simulink model "FOC_Compatible"  (R2020a)
settings: Solver=VariableStepAuto  StartTime=0.0  StopTime=10  MaxStep=0.0001  RelTol=1e-3
values from neighbouring files (symbols this model uses):
  B = [B1; zeros(2, 2)]    [LIM.m]
  D = [zeros(1, 2); zeros(1, 2 )]    [LIM.m]
undefined symbols (not defined in the file or in its folder): k, Ll, Lm, Lp, M, P, Rl, Rp, Tp
libraries: eeTransforms x2, simulink_extras x1, simulink x1
settings Model: Creator=Basilisk  LastModifiedBy=Basilisk
settings DebuggingCC: SFMachineParentedDataDiag=error

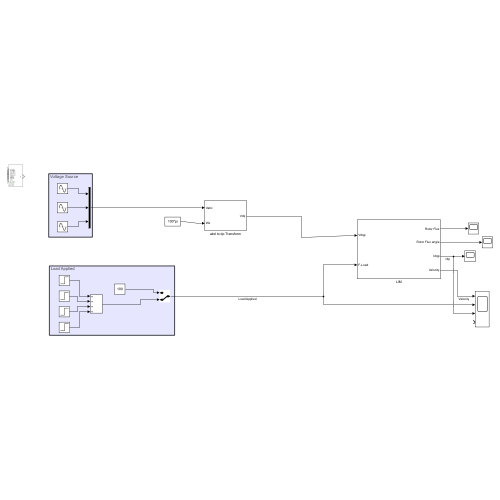
[thumbnail: Simulink's stored preview of the top-level diagram]
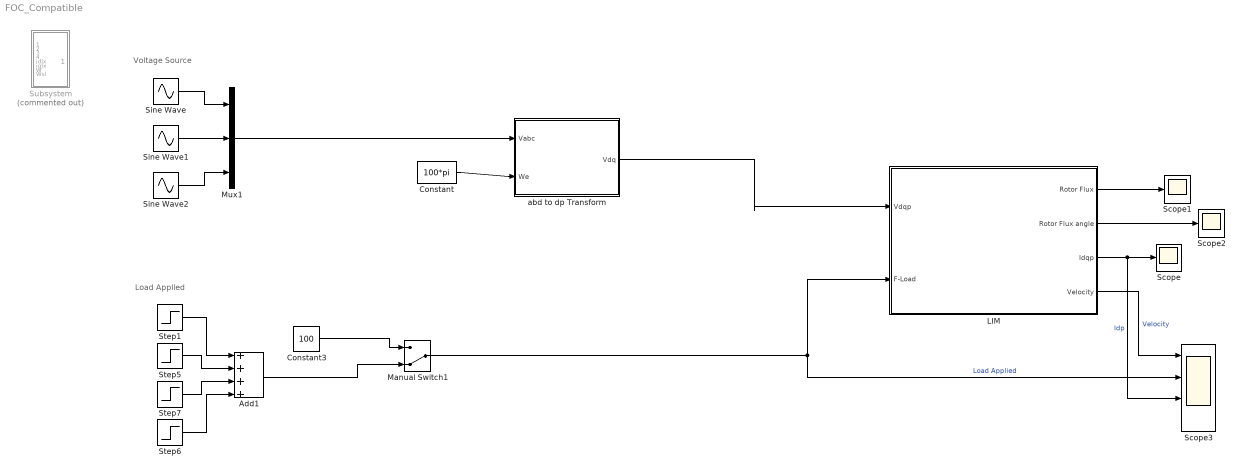
== system FOC_Compatible ==
  note: Load Applied
  note: Voltage Source
  Add1 : Sum  Inputs=++++
  Constant : Constant  Value=100*pi
  Constant3 : Constant  Value=100
  LIM : Subsystem
  Manual Switch1 : ManualSwitch  CurrentSetting=0
  Mux1 : Mux  Inputs=3
  Scope : Scope
  Scope1 : Scope
  Scope2 : Scope
  Scope3 : Scope  NumInputPorts=4
  Sine Wave : Sin  Amplitude=230  Frequency=100*pi  SampleTime=0
  Sine Wave1 : Sin  Amplitude=230  Frequency=100*pi  Phase=2*pi/3  SampleTime=0
  Sine Wave2 : Sin  Amplitude=230  Frequency=100*pi  Phase=-2*pi/3  SampleTime=0
  Step1 : Step  Time=0.5  After=4  SampleTime=0
  Step5 : Step  Time=0.9  After=50  SampleTime=0
  Step6 : Step  Time=2  After=50  SampleTime=0
  Step7 : Step  Time=1.5  After=100  SampleTime=0
  Subsystem : Subsystem  Commented=on
  abd to dp Transform : Subsystem
  wires:
  Step1/1 -> Add1/1
  Step7/1 -> Add1/3
  Step5/1 -> Add1/2
  Constant3/1 -> Manual Switch1/1
  Step6/1 -> Add1/4
  Add1/1 -> Manual Switch1/2
  Sine Wave1/1 -> Mux1/2
  Sine Wave/1 -> Mux1/1
  Sine Wave2/1 -> Mux1/3
  Mux1/1 -> abd to dp Transform/1(Vabc)
  Manual Switch1/1 -> LIM/2(F-Load), Scope3/2  "Load Applied"
  Constant/1 -> abd to dp Transform/2(We)
  LIM/3(Idqp) -> Scope3/3, Scope/1  "Idp"
  LIM/1(Rotor Flux) -> Scope1/1
  LIM/2(Rotor Flux angle) -> Scope2/1
  abd to dp Transform/1(Vdq) -> LIM/1(Vdqp)
  LIM/4(Velocity) -> Scope3/1  "Velocity"

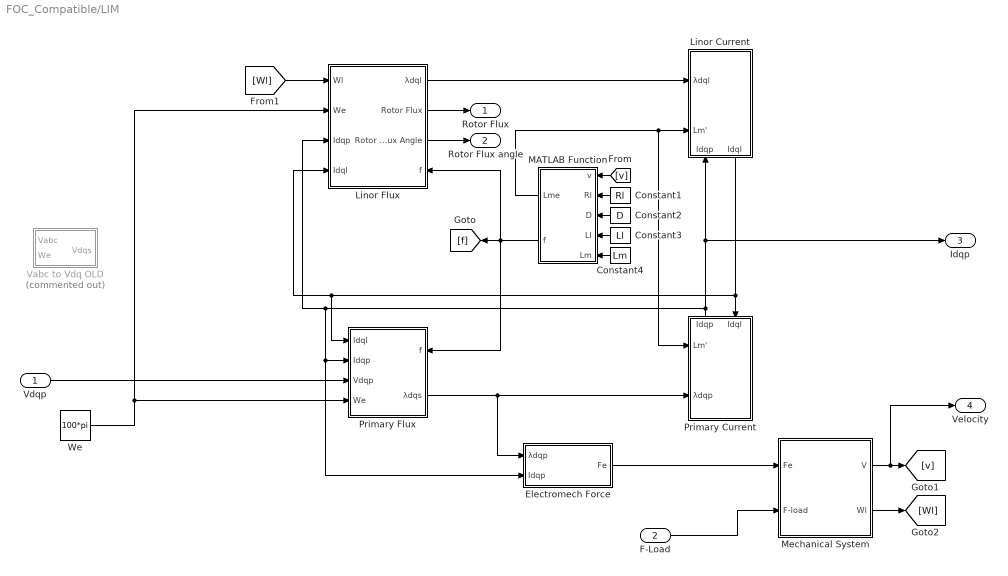
== system FOC_Compatible/LIM ==
  Vdqp : Inport
  F-Load : Inport  Port=2
  Constant1 : Constant  Value=Rl
  Constant2 : Constant  Value=D
  Constant3 : Constant  Value=Ll
  Constant4 : Constant  Value=Lm
  Electromech Force : Subsystem
  Linor Current : Subsystem
      settings: PortSchema="{\"entries\":[{\"content\":{\"sides\":[{\"content\":{\"connectorIds\":[\"In1\",\"In2\"]},\"type\":\"ConnectorPlacement.EquallySpacedRectSide\",\"uuid\":\"40d9865c-3cfa-44c1-93eb-682b1c6628f3\"},{\"content\":{\"connectorIds\":[],\"side\":\"RIGHT\"},\"type\":\"ConnectorPlacement.EquallySpacedRectSide\",\"uuid\":\"35710d59-e170-4e3b-9d71-9b17ce19d5d9\"},{\"content\":{\"connectorIds\":[],\"side\":\"TOP\"},\"type\":\"ConnectorPlacement.EquallySpacedRectSide\",\"uuid\":\"24aa0d2b-de57-4aff-b066-c7bd8ef57638\"},{\"content\":{\"connectorIds\":[\"In3\",\"Out1\"],\"side\":\"BOTTOM\"},\"type\":\"ConnectorPlacement.EquallySpacedRectSide\",\"uuid\":\"ba21e6b6-d163-44f4-8ede-2a2a18cab7d2\"}]},\"type\":\"ConnectorPlacement.EquallySpacedConnector\",\"uuid\":\"7a74cd09-26a1-4394-b388-2a31d7083798\"}],\"packageUris\":[\"http://schema.mathworks.com/mf0/Connector/R2020b\"],\"version\":\"1.0\"}"
  Linor Flux : Subsystem
      settings: PortSchema="{\"entries\":[{\"content\":{\"sides\":[{\"content\":{\"connectorIds\":[\"In1\",\"In2\",\"In3\",\"In4\"]},\"type\":\"ConnectorPlacement.EquallySpacedRectSide\",\"uuid\":\"b9a9f404-9b3b-4182-a50e-1bf7cef191e8\"},{\"content\":{\"connectorIds\":[\"Out1\",\"Out2\",\"Out3\",\"In5\"],\"side\":\"RIGHT\"},\"type\":\"ConnectorPlacement.EquallySpacedRectSide\",\"uuid\":\"68159d79-7975-4fd0-98a3-7e35432781a2\"},{\"content\":{\"connectorIds\":[],\"side\":\"TOP\"},\"type\":\"ConnectorPlacement.EquallySpacedRectSide\",\"uuid\":\"0c4dbb5d-b4d4-4876-b829-49090bd6eeb8\"}]},\"type\":\"ConnectorPlacement.EquallySpacedConnector\",\"uuid\":\"744eb17f-cf6a-4151-90db-78263b57d619\"}],\"packageUris\":[\"http://schema.mathworks.com/mf0/Connector/R2020b\"],\"version\":\"1.0\"}"
  MATLAB Function : MATLAB Function  TreatAsAtomicUnit=on
  Mechanical System : Subsystem
  Primary Current : Subsystem
      settings: PortSchema="{\"entries\":[{\"content\":{\"sides\":[{\"content\":{\"connectorIds\":[\"In1\",\"In2\"]},\"type\":\"ConnectorPlacement.EquallySpacedRectSide\",\"uuid\":\"40d9865c-3cfa-44c1-93eb-682b1c6628f3\"},{\"content\":{\"connectorIds\":[],\"side\":\"RIGHT\"},\"type\":\"ConnectorPlacement.EquallySpacedRectSide\",\"uuid\":\"35710d59-e170-4e3b-9d71-9b17ce19d5d9\"},{\"content\":{\"connectorIds\":[\"Out1\",\"In3\"],\"side\":\"TOP\"},\"type\":\"ConnectorPlacement.EquallySpacedRectSide\",\"uuid\":\"24aa0d2b-de57-4aff-b066-c7bd8ef57638\"}]},\"type\":\"ConnectorPlacement.EquallySpacedConnector\",\"uuid\":\"7a74cd09-26a1-4394-b388-2a31d7083798\"}],\"packageUris\":[\"http://schema.mathworks.com/mf0/Connector/R2020b\"],\"version\":\"1.0\"}"
  Primary Flux : Subsystem
      settings: PortSchema="{\"entries\":[{\"content\":{\"sides\":[{\"content\":{\"connectorIds\":[\"In1\",\"In2\",\"In3\",\"In4\"]},\"type\":\"ConnectorPlacement.EquallySpacedRectSide\",\"uuid\":\"a4b29cca-9cb0-4324-9244-2049ffc93668\"},{\"content\":{\"connectorIds\":[\"In5\",\"Out1\"],\"side\":\"RIGHT\"},\"type\":\"ConnectorPlacement.EquallySpacedRectSide\",\"uuid\":\"b20ff3ac-d40e-4f59-bb91-f6f2c0c6ca63\"},{\"content\":{\"connectorIds\":[],\"side\":\"TOP\"},\"type\":\"ConnectorPlacement.EquallySpacedRectSide\",\"uuid\":\"55342d43-b8f9-4aa9-846c-26670e92f4ca\"}]},\"type\":\"ConnectorPlacement.EquallySpacedConnector\",\"uuid\":\"78d5652d-2b6b-4c50-974b-d09ad892483f\"}],\"packageUris\":[\"http://schema.mathworks.com/mf0/Connector/R2020b\"],\"version\":\"1.0\"}"
  "Vabc to Vdq OLD " : Subsystem  Commented=on
  We : Constant  Value=100*pi
  Rotor Flux : Outport
  Rotor Flux angle : Outport  Port=2
  Idqp : Outport  Port=3
  Velocity : Outport  Port=4
  wires:
  Primary Flux/1(λdqs) -> Electromech Force/1(λdqp), Primary Current/2(λdqp)
  Vdqp/1 -> Primary Flux/3(Vdqp)
  Linor Flux/3(Rotor Flux Angle) -> Rotor Flux angle/1
  [v] -> MATLAB Function/1(v)
  Constant3/1 -> MATLAB Function/4(Ll)
  Constant2/1 -> MATLAB Function/3(D)
  Constant4/1 -> MATLAB Function/5(Lm)
  Constant1/1 -> MATLAB Function/2(Rl)
  MATLAB Function/2(f) -> Primary Flux/5(f), [f], Linor Flux/5(f)
  Linor Flux/1(λdql) -> Linor Current/1(λdql)
  MATLAB Function/1(Lme) -> Primary Current/1(Lm'), Linor Current/2(Lm')
  Linor Current/1(Idql) -> Primary Flux/1(Idql), Linor Flux/4(Idql), Primary Current/3(Idql)
  Primary Current/1(Idqp) -> Idqp/1, Linor Current/3(Idqp), Electromech Force/2(Idqp), Primary Flux/2(Idqp), Linor Flux/3(Idqp)
  Linor Flux/2(Rotor Flux) -> Rotor Flux/1
  Electromech Force/1(Fe) -> Mechanical System/1(Fe)
  F-Load/1 -> Mechanical System/2(F-load)
  Mechanical System/1(V) -> Velocity/1, [v]
  Mechanical System/2(Wl) -> [Wl]
  [Wl] -> Linor Flux/1(Wl)
  We/1 -> Linor Flux/2(We), Primary Flux/4(We)

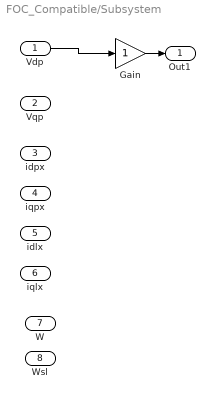
== system FOC_Compatible/Subsystem ==
  Vdp : Inport
  Vqp : Inport  Port=2
  idpx : Inport  Port=3
  iqpx : Inport  Port=4
  idlx : Inport  Port=5
  iqlx : Inport  Port=6
  W : Inport  Port=7
  Wsl : Inport  Port=8
  Gain : Gain
  Out1 : Outport
  wires:
  Vdp/1 -> Gain/1
  Gain/1 -> Out1/1

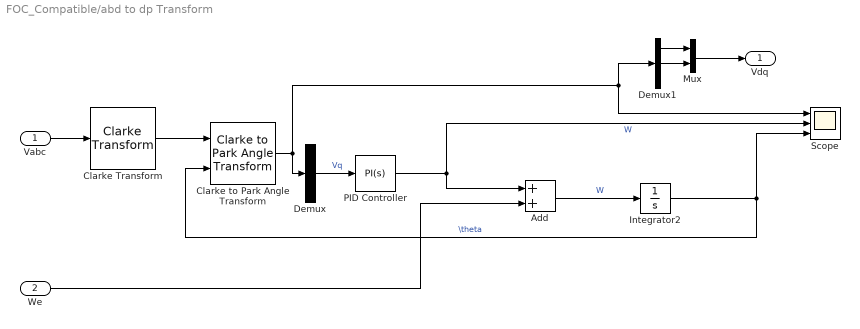
== system FOC_Compatible/abd to dp Transform ==
  Vabc : Inport
  We : Inport  Port=2
  Add : Sum
  Clarke Transform : eeTransforms/Clarke Transform  PowerInvariant=off
      settings: SourceProductBaseCode=PS
  Clarke to Park Angle Transform : eeTransforms/Clarke to Park Angle Transform  AxisAlignment=Q-axis
      settings: SourceProductBaseCode=PS
  Demux : Demux  Outputs=3
  Demux1 : Demux  Outputs=3
  Integrator2 : Integrator
  Mux : Mux  Inputs=2
  PID Controller : simulink/Continuous/PID Controller  Controller=PI  Form=Parallel  TimeDomain=Continuous-time  UseExternalTs=off  SampleTime=-1  IntegratorMethod=Forward Euler  FilterMethod=Forward Euler  ControllerParametersSource=internal  P=5  I=50  D=0  UseFilter=on  N=100  TunerSelectOption=Transfer Function Based (PID Tuner App)  InitialConditionSource=internal  InitialConditionForIntegrator=0  InitialConditionForFilter=0  DifferentiatorICPrevScaledInput=0  ExternalReset=none  TrackingMode=off  Kt=1  LimitOutput=off  UpperSaturationLimit=inf  LowerSaturationLimit=-inf  LinearizeAsGain=on  AntiWindupMode=none  Kb=1  POutMin=[]  POutMax=[]  IOutMin=[]  IOutMax=[]  DOutMin=[]  DOutMax=[]  NOutMin=[]  NOutMax=[]  SumOutMin=[]  SumOutMax=[]  SaturationOutMin=[]  SaturationOutMax=[]  PParamMin=[]  PParamMax=[]  IParamMin=[]  IParamMax=[]  DParamMin=[]  DParamMax=[]  NParamMin=[]  NParamMax=[]  KbParamMin=[]  KbParamMax=[]  KtParamMin=[]  KtParamMax=[]  KbOutMin=[]  KbOutMax=[]  KtOutMin=[]  KtOutMax=[]  IntegratorOutMin=[]  IntegratorOutMax=[]  FilterOutMin=[]  FilterOutMax=[]  SumI1OutMin=[]  SumI1OutMax=[]  SumI2OutMin=[]  SumI2OutMax=[]  SumI3OutMin=[]  SumI3OutMax=[]  SumI4OutMin=[]  SumI4OutMax=[]  SumDOutMin=[]  SumDOutMax=[]  DifferentiatorOutMin=[]  DifferentiatorOutMax=[]  FilterDiffOutCoefMin=[]  FilterDiffOutCoefMax=[]  ReciprocalOutMin=[]  ReciprocalOutMax=[]  SumDenOutMin=[]  SumDenOutMax=[]  SumNumOutMin=[]  SumNumOutMax=[]  DivideOutMin=[]  DivideOutMax=[]  UdiffTsProdOutMin=[]  UdiffTsProdOutMax=[]  NTsProdOutMin=[]  NTsProdOutMax=[]  UintegralTsProdOutMin=[]  UintegralTsProdOutMax=[]  UngainTsProdOutMin=[]  UngainTsProdOutMax=[]  IntegratorContinuousStateAttributes=''  IntegratorStateMustResolveToSignalObject=off  IntegratorRTWStateStorageClass=Auto  FilterContinuousStateAttributes=''  FilterStateMustResolveToSignalObject=off  FilterRTWStateStorageClass=Auto  ParallelPVariant=InternalParameters  IdealPVariant=Disabled  IVariant=InternalParameters  DVariant=Disabled  IntegratorVariant=Continuous  SatVariant=Disabled  AWVariant=Passthrough  PCopyVariant=Disabled  TRVariant=Disabled  FdbkBlocksVariant=Forward  IdealPFdbkVariant=Disabled  SatFdbkVariant=Disabled  DerivativeFilterVariant=Disabled  NVariant=Disabled  NCopyVariant=Disabled_SignalSpec  FilterICVariant=Disabled  IntegratorICVariant=InternalICs  ExternalResetVariant=Disabled  TRSumVariant=Passthrough  SumFdbkVariant=Disabled  SumVariant=Sum_PI  TsampFilterVariant=InternalTs  TsampNgainVariant=Passthrough  TsampIntegralVariant=Passthrough
  Scope : Scope  NumInputPorts=3
  Vdq : Outport
  wires:
  Integrator2/1 -> Scope/3, Clarke to Park Angle Transform/2  "\\theta"
  Clarke Transform/1 -> Clarke to Park Angle Transform/1
  Clarke to Park Angle Transform/1 -> Scope/1, Demux1/1, Demux/1
  We/1 -> Add/2
  Demux/2 -> PID Controller/1  "Vq"
  PID Controller/1 -> Scope/2, Add/1  "W"
  Add/1 -> Integrator2/1  "W"
  Vabc/1 -> Clarke Transform/1
  Mux/1 -> Vdq/1
  Demux1/2 -> Mux/2
  Demux1/1 -> Mux/1

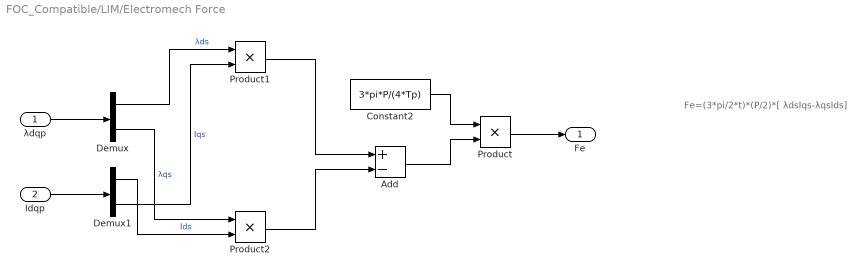
== system FOC_Compatible/LIM/Electromech Force ==
  note: Fe=(3*pi/2*t)*(P/2)*[ λdsIqs-λqsIds]
  λdqp : Inport
  Idqp : Inport  Port=2
  Add : Sum  Inputs=+-
  Constant2 : Constant  Value=3*pi*P/(4*Tp)
  Demux : Demux  Outputs=2
  Demux1 : Demux  Outputs=2
  Product : Product
  Product1 : Product
  Product2 : Product
  Fe : Outport
  wires:
  Product/1 -> Fe/1
  λdqp/1 -> Demux/1
  Idqp/1 -> Demux1/1
  Add/1 -> Product/2
  Demux/1 -> Product1/1  "λds"
  Demux1/2 -> Product1/2  "Iqs"
  Demux/2 -> Product2/1  "λqs"
  Demux1/1 -> Product2/2  "Ids"
  Product1/1 -> Add/1
  Product2/1 -> Add/2
  Constant2/1 -> Product/1

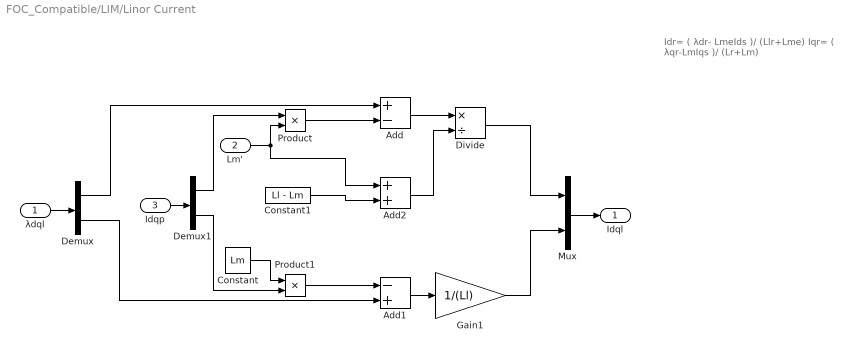
== system FOC_Compatible/LIM/Linor Current ==
  note: Idr= ( λdr- LmeIds )/ (Llr+Lme)
      |
      | Iqr= ( λqr-LmIqs )/ (Lr+Lm)
  λdql : Inport
  Lm' : Inport  Port=2
  Idqp : Inport  Port=3
  Add : Sum  Inputs=+-
  Add1 : Sum  Inputs=-+
  Add2 : Sum
  Constant : Constant  Value=Lm  VectorParams1D=off
  Constant1 : Constant  Value=Ll - Lm
  Demux : Demux  Outputs=2
  Demux1 : Demux  Outputs=2
  Divide : Product  Inputs=*/
  Gain1 : Gain  Gain=1/(Ll)
  Mux : Mux  Inputs=2
  Product : Product
  Product1 : Product
  Idql : Outport
  wires:
  Mux/1 -> Idql/1
  λdql/1 -> Demux/1
  Idqp/1 -> Demux1/1
  Demux1/1 -> Product/1
  Demux1/2 -> Product1/2
  Demux/1 -> Add/1
  Demux/2 -> Add1/2
  Product/1 -> Add/2
  Product1/1 -> Add1/1
  Add/1 -> Divide/1
  Add1/1 -> Gain1/1
  Gain1/1 -> Mux/2
  Divide/1 -> Mux/1
  Constant/1 -> Product1/1
  Constant1/1 -> Add2/2
  Lm'/1 -> Add2/1, Product/2
  Add2/1 -> Divide/2

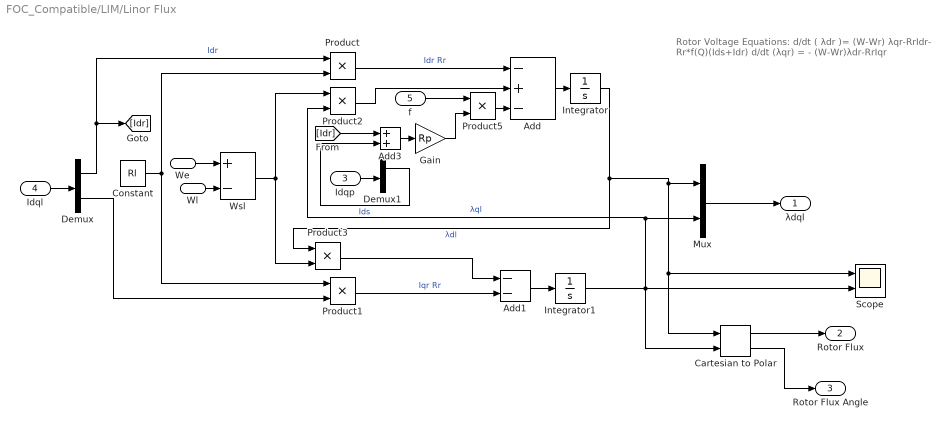
== system FOC_Compatible/LIM/Linor Flux ==
  note: Rotor Voltage Equations:
      | d/dt ( λdr )= (W-Wr) λqr-RrIdr- Rr*f(Q)(Ids+Idr)
      | d/dt (λqr) = - (W-Wr)λdr-RrIqr
  Wl : Inport
  We : Inport  Port=2
  Idqp : Inport  Port=3
  Idql : Inport  Port=4
  f : Inport  Port=5
  Add : Sum  Inputs=-+-
  Add1 : Sum  Inputs=--
  Add3 : Sum
  Cartesian to Polar : simulink_extras/Transformations/Cartesian to Polar
  Constant : Constant  Value=Rl
  Demux : Demux  Outputs=2
  Demux1 : Demux  Outputs=2
  Gain : Gain  Gain=Rp
  Integrator : Integrator
  Integrator1 : Integrator
  Mux : Mux  Inputs=2
  Product{,1..3,5} (5 alike) : Product
  Scope : Scope  NumInputPorts=2
  Wsl : Sum  Inputs=+-
  λdql : Outport
  Rotor Flux : Outport  Port=2
  Rotor Flux Angle : Outport  Port=3
  wires:
  Mux/1 -> λdql/1
  Idql/1 -> Demux/1
  Demux/1 -> [Idr], Product/1  "Idr"
  Demux/2 -> Product1/2
  Constant/1 -> Product1/1, Product/2
  Product/1 -> Add/1  "Idr Rr"
  Product1/1 -> Add1/2  "Iqr Rr"
  Add/1 -> Integrator/1
  Add1/1 -> Integrator1/1
  We/1 -> Wsl/1
  Wl/1 -> Wsl/2
  Wsl/1 -> Product3/2, Product2/1
  Product2/1 -> Add/2
  Product3/1 -> Add1/1
  Demux1/1 -> Add3/2  "Ids"
  Product5/1 -> Add/3
  Add3/1 -> Gain/1
  Gain/1 -> Product5/2
  f/1 -> Product5/1
  Idqp/1 -> Demux1/1
  [Idr] -> Add3/1
  Cartesian to Polar/1 -> Rotor Flux/1
  Cartesian to Polar/2 -> Rotor Flux Angle/1
  Integrator1/1 -> Product2/2, Mux/2, Scope/2, Cartesian to Polar/2  "λql"
  Integrator/1 -> Product3/1, Cartesian to Polar/1, Scope/1, Mux/1  "λdl"

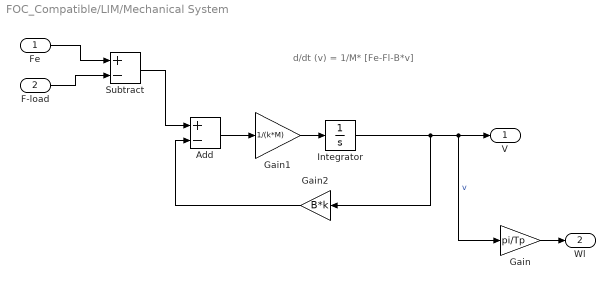
== system FOC_Compatible/LIM/Mechanical System ==
  note: d/dt (v) = 1/M* [Fe-Fl-B*v]
  Fe : Inport
  F-load : Inport  Port=2
  Add : Sum  Inputs=+-
  Gain : Gain  Gain=pi/Tp
  Gain1 : Gain  Gain=1/(k*M)
  Gain2 : Gain  Gain=B*k
  Integrator : Integrator
  Subtract : Sum  Inputs=+-
  V : Outport
  Wl : Outport  Port=2
  wires:
  Fe/1 -> Subtract/1
  F-load/1 -> Subtract/2
  Gain/1 -> Wl/1
  Subtract/1 -> Add/1
  Gain1/1 -> Integrator/1
  Integrator/1 -> Gain/1, V/1, Gain2/1  "v"
  Add/1 -> Gain1/1
  Gain2/1 -> Add/2

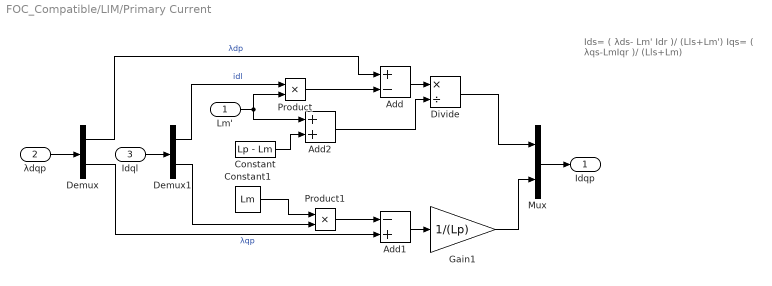
== system FOC_Compatible/LIM/Primary Current ==
  note: Ids= ( λds- Lm' Idr )/ (Lls+Lm')
      |
      | Iqs= ( λqs-LmIqr )/ (Lls+Lm)
  Lm' : Inport
  λdqp : Inport  Port=2
  Idql : Inport  Port=3
  Add : Sum  Inputs=+-
  Add1 : Sum  Inputs=-+
  Add2 : Sum
  Constant : Constant  Value=Lp - Lm
  Constant1 : Constant  Value=Lm  VectorParams1D=off
  Demux : Demux  Outputs=2
  Demux1 : Demux  Outputs=2
  Divide : Product  Inputs=*/
  Gain1 : Gain  Gain=1/(Lp)
  Mux : Mux  Inputs=2
  Product : Product
  Product1 : Product
  Idqp : Outport
  wires:
  Demux/2 -> Add1/2  "λqp"
  Demux1/1 -> Product/1  "idl"
  Product/1 -> Add/2
  Product1/1 -> Add1/1
  λdqp/1 -> Demux/1
  Add1/1 -> Gain1/1
  Mux/1 -> Idqp/1
  Idql/1 -> Demux1/1
  Demux/1 -> Add/1  "λdp"
  Demux1/2 -> Product1/2
  Add/1 -> Divide/1
  Divide/1 -> Mux/1
  Gain1/1 -> Mux/2
  Constant1/1 -> Product1/1
  Lm'/1 -> Add2/1, Product/2
  Constant/1 -> Add2/2
  Add2/1 -> Divide/2

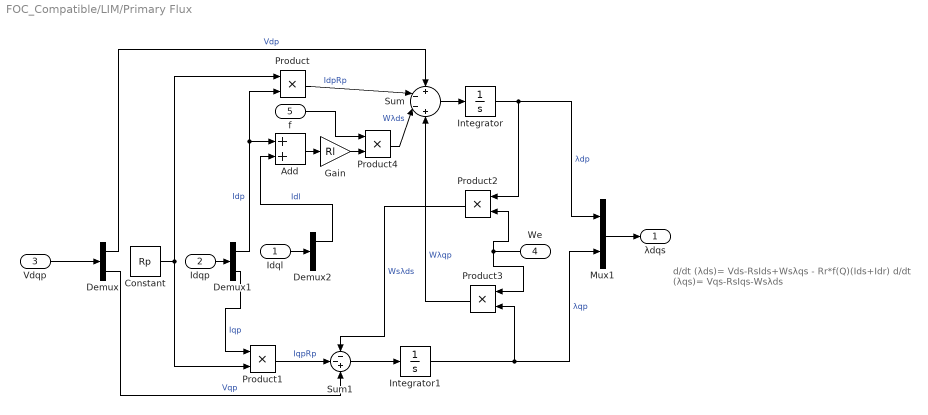
== system FOC_Compatible/LIM/Primary Flux ==
  note: d/dt (λds)= Vds-RsIds+Wsλqs - Rr*f(Q)(Ids+Idr)
      |
      | d/dt (λqs)= Vqs-RsIqs-Wsλds
  Idql : Inport
  Idqp : Inport  Port=2
  Vdqp : Inport  Port=3
  We : Inport  Port=4
  f : Inport  Port=5
  Add : Sum
  Constant : Constant  Value=Rp
  Demux : Demux  Outputs=2
  Demux1 : Demux  Outputs=2
  Demux2 : Demux  Outputs=2
  Gain : Gain  Gain=Rl
  Integrator : Integrator
  Integrator1 : Integrator
  Mux1 : Mux  Inputs=2
  Product{,1..4} (5 alike) : Product
  Sum : Sum  Inputs=+--+
  Sum1 : Sum  Inputs=--+
  λdqs : Outport
  wires:
  Integrator1/1 -> Product3/2, Mux1/2  "λqp"
  Integrator/1 -> Product2/1, Mux1/1  "λdp"
  Vdqp/1 -> Demux/1
  Idqp/1 -> Demux1/1
  Demux/1 -> Sum/1  "Vdp"
  Sum/1 -> Integrator/1
  Constant/1 -> Product1/2, Product/1
  Demux1/1 -> Product/2, Add/1  "Idp"
  Product/1 -> Sum/2  "IdpRp"
  Sum1/1 -> Integrator1/1
  Demux/2 -> Sum1/3  "Vqp"
  Demux1/2 -> Product1/1  "Iqp"
  Product1/1 -> Sum1/2  "IqpRp"
  We/1 -> Product3/1, Product2/2
  Product3/1 -> Sum/4  "Wλqp"
  Product2/1 -> Sum1/1  "Wsλds"
  Mux1/1 -> λdqs/1
  Idql/1 -> Demux2/1
  Demux2/1 -> Add/2  "Idl"
  Add/1 -> Gain/1
  Gain/1 -> Product4/2
  Product4/1 -> Sum/3  "Wλds"
  f/1 -> Product4/1

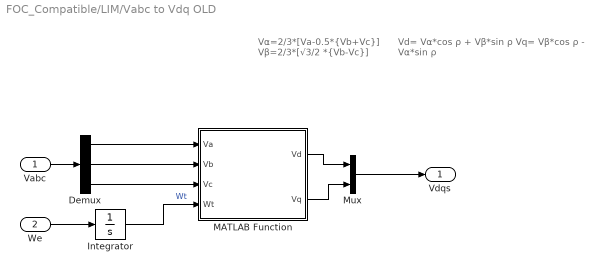
== system FOC_Compatible/LIM/Vabc to Vdq OLD  ==
  note: Vα=2/3*[Va-0.5*{Vb+Vc}]
      |
      | Vβ=2/3*[√3/2 *{Vb-Vc}]
  note: Vd= Vα*cos ρ + Vβ*sin ρ
      |
      | Vq= Vβ*cos ρ - Vα*sin ρ
  Vabc : Inport
  We : Inport  Port=2
  Demux : Demux  Outputs=3
  Integrator : Integrator
  MATLAB Function : MATLAB Function  TreatAsAtomicUnit=on
  Mux : Mux  Inputs=2
  Vdqs : Outport
  wires:
  Vabc/1 -> Demux/1
  Demux/1 -> MATLAB Function/1(Va)
  Demux/2 -> MATLAB Function/2(Vb)
  Demux/3 -> MATLAB Function/3(Vc)
  We/1 -> Integrator/1
  Integrator/1 -> MATLAB Function/4(Wt)  "Wt"
  Mux/1 -> Vdqs/1
  MATLAB Function/1(Vd) -> Mux/1
  MATLAB Function/2(Vq) -> Mux/2

== matlab function FOC_Compatible/LIM/Vabc to Vdq OLD /MATLAB Function ==
  data: Va input; Vd output; Vb input; Vc input; Wt input; Vq output
function [Vd,Vq] = Transform(Va, Vb, Vc, Wt)
    M = [cos(Wt)    cos(Wt - 2*pi/3)    cos(Wt-4*pi/3);
        -sin(Wt)    -sin(Wt- 2*pi/3)    -sin(Wt-4*pi/3);
        1/sqrt(2)       1/sqrt(2)           1/sqrt(2)];
    
    DQ = M*[Va,Vb,Vc]';
    
    Vd = DQ(1);
    Vq = DQ(2);
end

== matlab function FOC_Compatible/LIM/MATLAB Function ==
  data: v input; Lme output; Rl input; D input; Ll input; Lm input; f output
function [Lme,f]= fcn(v, Rl,D,Ll,Lm)
Q=abs((D*Rl)/(Ll*v));

f=(1-(exp(-Q)))/Q;

Lme = Lm*(1-f);
